simulink model "HW_1"  (R2023a)
settings: Solver=VariableStepAuto  StartTime=0.0  StopTime=70  RelTol=1e-3
libraries: simulink x1
settings Model: Creator=ПК  LastModifiedBy=ПК

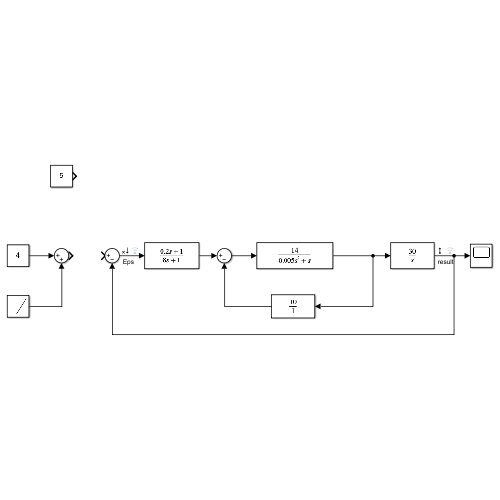
[thumbnail: Simulink's stored preview of the top-level diagram]
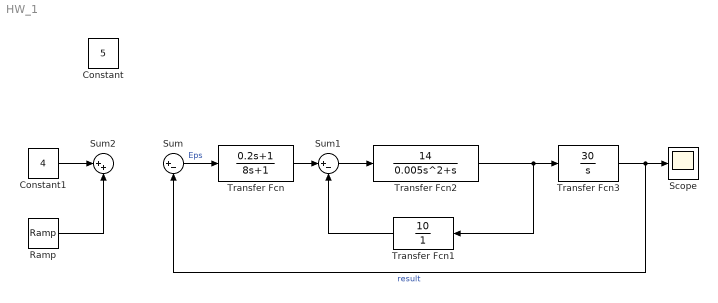
== system HW_1 ==
  Constant : Constant  Value=5
  Constant1 : Constant  Value=4
  Ramp : simulink/Sources/Ramp  slope=0.5  start=0  InitialOutput=0
  Scope : Scope
  Sum : Sum  Inputs=|+-
  Sum1 : Sum  Inputs=|+-
  Sum2 : Sum  Inputs=|++
  Transfer Fcn : TransferFcn  Numerator=[0.2 1]  Denominator=[8 1]
  Transfer Fcn1 : TransferFcn  Numerator=[10]  Denominator=[1]
  Transfer Fcn2 : TransferFcn  Numerator=[14]  Denominator=[0.005 1 0]
  Transfer Fcn3 : TransferFcn  Numerator=[30]  Denominator=[1 0]
  wires:
  Transfer Fcn3/1 -> Sum/2, Scope/1  "result"
  Sum/1 -> Transfer Fcn/1  "Eps"
  Transfer Fcn/1 -> Sum1/1
  Transfer Fcn2/1 -> Transfer Fcn1/1, Transfer Fcn3/1
  Transfer Fcn1/1 -> Sum1/2
  Sum1/1 -> Transfer Fcn2/1
  Constant1/1 -> Sum2/1
  Ramp/1 -> Sum2/2
